simulink model "OPENXWD"  (R2021b)
settings: Solver=ode45  StartTime=0.0  StopTime=inf  RelTol=1e-3  EnableMultiTasking=on
PreLoadFcn:
  | run('Parameters\FSE_Parameters.m')
undefined symbols (not defined in the file): i_Diff
libraries: simulink x28, CarMaker4SL x17, eeGeneralControl x6
(part 3 of 8)

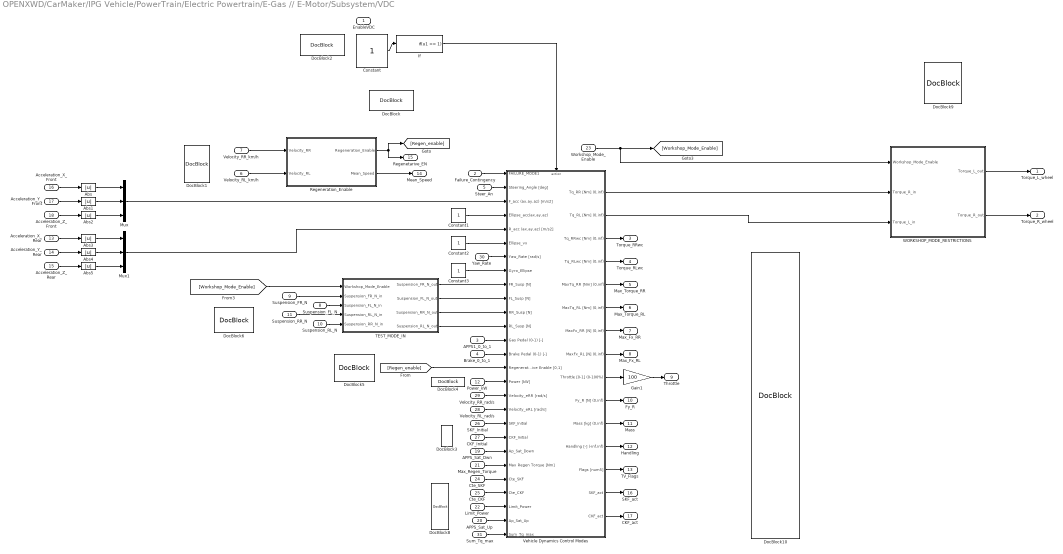
== system OPENXWD/CarMaker/IPG Vehicle/PowerTrain/Electric Powertrain/E-Gas // E-Motor/Subsystem/VDC ==
  EnableVDC : Inport
  Failure_Contingency : Inport  Port=2
  APPS1_0_to_1 : Inport  Port=3
  Brake_0_to_1 : Inport  Port=4
  Steer_An : Inport  Port=5
  Velocity_RL_km/h : Inport  Port=6
  Velocity_RR_km/h : Inport  Port=7
  Suspension_FL_N : Inport  Port=8
  Suspension_FR_N : Inport  Port=9
  Suspension_RL_N : Inport  Port=10
  Suspension_RR_N : Inport  Port=11
  Power_kW : Inport  Port=12
  Acceleration_X_Rear : Inport  Port=13
  Acceleration_Y_Rear : Inport  Port=14
  Acceleration_Z_Rear : Inport  Port=15
  Acceleration_X_Front : Inport  Port=16
  Acceleration_Y_Front : Inport  Port=17
  Acceleration_Z_Front : Inport  Port=18
  APPS_Sat_Dwn : Inport  Port=19
  APPS_Sat_Up : Inport  Port=20
  Max_Regen_Torque : Inport  Port=21
  Limit_Power : Inport  Port=22
  Workshop_Mode_Enable : Inport  Port=23
  Cte_SKF : Inport  Port=24
  Cte_CKF : Inport  Port=25
  SKF_Initial : Inport  Port=26
  CKF_Initial : Inport  Port=27
  Velocity_RL_rad/s : Inport  Port=28
  Velocity_RR_rad/s : Inport  Port=29
  Yaw_Rate : Inport  Port=30
  Sum_Tq_max : Inport  Port=31
  Abs{,1..5} (6 alike) : Abs
  Constant{,1..3} (4 alike) : Constant
  DocBlock{,1..6,8..10} (10 alike) : simulink/Model-Wide Utilities/DocBlock  DocumentType=Text
  Gain1 : Gain  Gain=100
  If : If  IfExpression=u1 == 1  ShowElse=off
  Mux : Mux  Inputs=3
  Mux1 : Mux  Inputs=3
  Regeneration_Enable : Subsystem  TreatAsAtomicUnit=on
  TEST_MODE_IN : Subsystem  TreatAsAtomicUnit=on
  Vehicle Dynamics Control Modes : Subsystem
  WORKSHOP_MODE_RESTRICTIONS : Subsystem  TreatAsAtomicUnit=on
  Torque_L_wheel : Outport  VectorParamsAs1DForOutWhenUnconnected=off
  Torque_R_wheel : Outport  Port=2  VectorParamsAs1DForOutWhenUnconnected=off
  Torque_RRwc : Outport  Port=3  VectorParamsAs1DForOutWhenUnconnected=off
  Torque_RLwc : Outport  Port=4  VectorParamsAs1DForOutWhenUnconnected=off
  Max_Torque_RR : Outport  Port=5  VectorParamsAs1DForOutWhenUnconnected=off
  Max_Torque_RL : Outport  Port=6  VectorParamsAs1DForOutWhenUnconnected=off
  Max_Fx_RR : Outport  Port=7  VectorParamsAs1DForOutWhenUnconnected=off
  Max_Fx_RL : Outport  Port=8  VectorParamsAs1DForOutWhenUnconnected=off
  Throttle : Outport  Port=9  VectorParamsAs1DForOutWhenUnconnected=off
  Fy_R : Outport  Port=10  VectorParamsAs1DForOutWhenUnconnected=off
  Mass : Outport  Port=11  VectorParamsAs1DForOutWhenUnconnected=off
  Handling : Outport  Port=12  VectorParamsAs1DForOutWhenUnconnected=off
  TV_Flags : Outport  Port=13  VectorParamsAs1DForOutWhenUnconnected=off
  Mean_Speed : Outport  Port=14  VectorParamsAs1DForOutWhenUnconnected=off
  Regenetarive_EN : Outport  Port=15  VectorParamsAs1DForOutWhenUnconnected=off
  SKF_act : Outport  Port=16  VectorParamsAs1DForOutWhenUnconnected=off
  CKF_act : Outport  Port=17  VectorParamsAs1DForOutWhenUnconnected=off
  wires:
  Velocity_RR_km/h/1 -> Regeneration_Enable/1(Velocity_RR)
  Acceleration_Z_Front/1 -> Abs2/1
  Abs2/1 -> Mux/3
  Gain1/1 -> Throttle/1
  Vehicle Dynamics Control Modes/7(MaxFx_RR [N] (0,inf)) -> Max_Fx_RR/1
  Vehicle Dynamics Control Modes/6(MaxTq_RL [Nm] (0,inf)) -> Max_Torque_RL/1
  Acceleration_X_Rear/1 -> Abs3/1
  Acceleration_Y_Front/1 -> Abs1/1
  Abs4/1 -> Mux1/2
  Vehicle Dynamics Control Modes/8(MaxFx_RL [N] (0,inf)) -> Max_Fx_RL/1
  Power_kW/1 -> Vehicle Dynamics Control Modes/16(Power [kW])
  Vehicle Dynamics Control Modes/1(Tq_RR [Nm] (0,inf)) -> WORKSHOP_MODE_RESTRICTIONS/2(Torque_R_in)
  Abs/1 -> Mux/1
  Abs5/1 -> Mux1/3
  Acceleration_Y_Rear/1 -> Abs4/1
  APPS_Sat_Up/1 -> Vehicle Dynamics Control Modes/26(Ap_Sat_Up)
  WORKSHOP_MODE_RESTRICTIONS/1(Torque_L_out) -> Torque_L_wheel/1
  Acceleration_Z_Rear/1 -> Abs5/1
  Vehicle Dynamics Control Modes/3(Tq_RRwc [Nm] (0,inf)) -> Torque_RRwc/1
  Suspension_FL_N/1 -> TEST_MODE_IN/3(Suspension_FL_N_in)
  Suspension_FR_N/1 -> TEST_MODE_IN/2(Suspension_FR_N_in)
  TEST_MODE_IN/1(Suspension_FR_N_out) -> Vehicle Dynamics Control Modes/9(FR_Susp [N])
  Velocity_RR_rad/s/1 -> Vehicle Dynamics Control Modes/17(Velocity_eRR [rad/s])
  Vehicle Dynamics Control Modes/14(SKF_act) -> SKF_act/1
  APPS1_0_to_1/1 -> Vehicle Dynamics Control Modes/13(Gas Pedal (0-1) [-])
  Vehicle Dynamics Control Modes/4(Tq_RLwc [Nm] (0,inf)) -> Torque_RLwc/1
  Vehicle Dynamics Control Modes/5(MaxTq_RR [Nm] (0,inf)) -> Max_Torque_RR/1
  Brake_0_to_1/1 -> Vehicle Dynamics Control Modes/14(Brake Pedal (0-1) [-])
  Velocity_RL_km/h/1 -> Regeneration_Enable/2(Velocity_RL)
  Vehicle Dynamics Control Modes/11(Mass [kg] (0,inf)) -> Mass/1
  Vehicle Dynamics Control Modes/9(Throttle [0-1] (0-100%)) -> Gain1/1
  Vehicle Dynamics Control Modes/2(Tq_RL [Nm] (0,inf)) -> WORKSHOP_MODE_RESTRICTIONS/3(Torque_L_in)
  Constant/1 -> If/1
  Regeneration_Enable/2(Mean_Speed) -> Mean_Speed/1
  Suspension_RL_N/1 -> TEST_MODE_IN/5(Suspension_RR_N_in)
  Vehicle Dynamics Control Modes/10(Fy_R [N] (0,inf)) -> Fy_R/1
  Vehicle Dynamics Control Modes/13(Flags [num5]) -> TV_Flags/1
  Abs1/1 -> Mux/2
  [Workshop_Mode_Enable] -> TEST_MODE_IN/1(Workshop_Mode_Enable)
  Acceleration_X_Front/1 -> Abs/1
  Abs3/1 -> Mux1/1
  Suspension_RR_N/1 -> TEST_MODE_IN/4(Suspension_RL_N_in)
  Vehicle Dynamics Control Modes/12(Handling [-] (-inf,inf)) -> Handling/1
  Workshop_Mode_Enable/1 -> [Workshop_Mode_Enable], WORKSHOP_MODE_RESTRICTIONS/1(Workshop_Mode_Enable)
  Vehicle Dynamics Control Modes/15(CKF_act) -> CKF_act/1
  If/1 -> Vehicle Dynamics Control Modes/Action
  TEST_MODE_IN/2(Suspension_FL_N_out) -> Vehicle Dynamics Control Modes/10(FL_Susp [N])
  TEST_MODE_IN/3(Suspension_RR_N_out) -> Vehicle Dynamics Control Modes/11(RR_Susp [N])
  TEST_MODE_IN/4(Suspension_RL_N_out) -> Vehicle Dynamics Control Modes/12(RL_Susp [N])
  Velocity_RL_rad/s/1 -> Vehicle Dynamics Control Modes/18(Velocity_eRL [rad/s])
  SKF_Initial/1 -> Vehicle Dynamics Control Modes/19(SKF_Initial)
  CKF_Initial/1 -> Vehicle Dynamics Control Modes/20(CKF_Initial)
  APPS_Sat_Dwn/1 -> Vehicle Dynamics Control Modes/21(Ap_Sat_Down)
  Max_Regen_Torque/1 -> Vehicle Dynamics Control Modes/22(Max Regen Torque [Nm])
  Cte_SKF/1 -> Vehicle Dynamics Control Modes/23(Cte_SKF)
  Cte_CKF/1 -> Vehicle Dynamics Control Modes/24(Cte_CKF)
  Steer_An/1 -> Vehicle Dynamics Control Modes/2(Steering_Angle [deg])
  Mux/1 -> Vehicle Dynamics Control Modes/3(F_acc (ax,ay,az) [m/s2])
  Mux1/1 -> Vehicle Dynamics Control Modes/5(R_acc (ax,ay,az) [m/s2])
  Failure_Contingency/1 -> Vehicle Dynamics Control Modes/1(FAILURE_MODE1)
  Constant1/1 -> Vehicle Dynamics Control Modes/4(Ellipse_acc(ax,ay,az))
  Constant2/1 -> Vehicle Dynamics Control Modes/6(Ellipse_vx)
  Yaw_Rate/1 -> Vehicle Dynamics Control Modes/7(Yaw_Rate [rad/s])
  Constant3/1 -> Vehicle Dynamics Control Modes/8(Gyro_Ellipse)
  Regeneration_Enable/1(Regeneration_Enable) -> Regenetarive_EN/1, [Regen_enable]
  [Regen_enable] -> Vehicle Dynamics Control Modes/15(Regenerative Enable [0,1])
  WORKSHOP_MODE_RESTRICTIONS/2(Torque_R_out) -> Torque_R_wheel/1
  Limit_Power/1 -> Vehicle Dynamics Control Modes/25(Limit_Power)
  Sum_Tq_max/1 -> Vehicle Dynamics Control Modes/27(Sum_Tq_max)

== system OPENXWD/CarMaker/IPG Vehicle/PowerTrain/Electric Powertrain/E-Gas // E-Motor/Subsystem/W to kW ==
  Power : Inport
  0-100 to 0-2 : Constant  Value=1000
  Divide5 : Product  Inputs=*/
  Out : Outport  VectorParamsAs1DForOutWhenUnconnected=off
  wires:
  Power/1 -> Divide5/1
  0-100 to 0-2/1 -> Divide5/2
  Divide5/1 -> Out/1

== system OPENXWD/CarMaker/IPG Vehicle/PowerTrain/Electric Powertrain/E-Gas // E-Motor/Subsystem/power_limitation1 ==
  note: Inputs:
      | max_cell_temp: signal from AMS_Master (Highest_Cell_Temp) [ºC]
      | max_inverter_temp: highest temperature of any of the inverters [ºC]
      | max_motor_temp: highest temperature of any of the motors [ºC]
      | SoC_Low, SoC_High: Lowest & Highest cell state of charge (0-100) [%]
  note: Outputs:
      | Flags: 1 means power is being limited by temperature, 0 means not limited
      | SoP_discharge: State of Power for discharging
      | SoP_charge: State of Power for charging
  max_motor_temp : Inport
  max_inverter_temp : Inport  Port=2
  max_cell_temp : Inport  Port=3
  SoC_Low : Inport  Port=4
  SoC_High : Inport  Port=5
  Saturation : Saturate  UpperLimit=1  LowerLimit=0
  Saturation1 : Saturate  UpperLimit=1  LowerLimit=0
  SoC_SoP : Subsystem
  initial_limitation : Constant  Value=0.4
  temperature_SoP : Subsystem
  Accu_Temperature_Limitation_Flag : Outport
  Inverters_Temperature_Limitation_Flag : Outport  Port=2
  Motors_Temperature_Limitation_Flag : Outport  Port=3
  SoP_Discharge : Outport  Port=4
  SoP_Regen : Outport  Port=5
  wires:
  SoC_SoP/1(SoP_Discharge) -> Saturation/1  "SoP_Discharge"
  SoC_SoP/2(SoP_Regen) -> Saturation1/1  "SoP_Regen"
  max_motor_temp/1 -> temperature_SoP/1(max_motor_temp)
  max_inverter_temp/1 -> temperature_SoP/2(max_inverter_temp)
  max_cell_temp/1 -> temperature_SoP/3(max_cell_temp), SoC_SoP/4(max_cell_temp)
  initial_limitation/1 -> temperature_SoP/4(initial_limitation)
  temperature_SoP/1(SoP) -> SoC_SoP/3(SoP_Temperature)  "temperature_SoP"
  temperature_SoP/4(Motors_Temperature_Limitation_Flag) -> Motors_Temperature_Limitation_Flag/1
  temperature_SoP/3(Inverters_Temperature_Limitation_Flag) -> Inverters_Temperature_Limitation_Flag/1
  temperature_SoP/2(Accu_Temperature_Limitation_Flag) -> Accu_Temperature_Limitation_Flag/1
  SoC_High/1 -> SoC_SoP/2(SoC_High)
  SoC_Low/1 -> SoC_SoP/1(SoC_Low)
  Saturation/1 -> SoP_Discharge/1
  Saturation1/1 -> SoP_Regen/1

== system OPENXWD/CarMaker/IPG Vehicle/PowerTrain/Electric Powertrain/E-Gas // E-Motor/Subsystem/Accumulator Power/PowerLimitDetection ==
  note: mean:500ms
      | time:25ms
      | moving window: 500/25=20
  Power : Inport
  Data Store Memory10 : DataStoreMemory  ReadBeforeWriteMsg=warning  WriteAfterWriteMsg=warning  WriteAfterReadMsg=warning  ShowAdditionalParam=off
  Data Store Read30 : DataStoreRead  IndexOptions=Index vector (dialog)  Indices=1  OutputSizes=1
  Data Store Write20 : DataStoreWrite  IndexOptions=Index vector (dialog)  Indices=1  OutputSizes=1
  If : If  IfExpression=u1 >= 80000
  LimitReached : Subsystem  TreatAsAtomicUnit=on
  Merge1 : Merge
  OK_OrLatch : Subsystem  TreatAsAtomicUnit=on
  PowerLimitReached : Outport  VectorParamsAs1DForOutWhenUnconnected=off
  PowerMean500ms : Outport  Port=2  VectorParamsAs1DForOutWhenUnconnected=off
  wires:
  Power/1 -> If/1, PowerMean500ms/1
  If/1 -> LimitReached/Action
  If/2 -> OK_OrLatch/Action
  LimitReached/1("Out ") -> Merge1/1
  OK_OrLatch/1(Out 1) -> Merge1/2
  Merge1/1 -> Data Store Write20/1, PowerLimitReached/1
  Data Store Read30/1 -> OK_OrLatch/1(IN)

== system OPENXWD/CarMaker/IPG Vehicle/PowerTrain/Electric Powertrain/E-Gas // E-Motor/Subsystem/Calculate Current Conversion/KT_L_TORKY ==
  Torque : Inport
  A/Nm : Gain  Gain=0.2
  Current : Outport  VectorParamsAs1DForOutWhenUnconnected=off
  wires:
  A/Nm/1 -> Current/1
  Torque/1 -> A/Nm/1

== system OPENXWD/CarMaker/IPG Vehicle/PowerTrain/Electric Powertrain/E-Gas // E-Motor/Subsystem/Calculate Current Conversion/KT_R_EMY ==
  Torque : Inport
  A/Nm : Gain  Gain=0.2
  Current : Outport  VectorParamsAs1DForOutWhenUnconnected=off
  wires:
  Torque/1 -> A/Nm/1
  A/Nm/1 -> Current/1

== system OPENXWD/CarMaker/IPG Vehicle/PowerTrain/Electric Powertrain/E-Gas // E-Motor/Subsystem/Controls Temperature by limiting Torque/SoC_SoP ==
  note: El lookup se puede obtener ensayando una celda en una descarga y en una carga con pérdidas de calor constantes. La corriente normalizada será el lookup.
  note: Si está descargada, no descargues más
  note: Si está cargada, no
      | cargues más
  SoC_Low : Inport
  SoC_High : Inport  Port=2
  SoP_Temperature : Inport  Port=3
  max_cell_temp : Inport  Port=4
  Gain5 : Gain  Gain=1/100
  Gain6 : Gain  Gain=1/100
  Lookup_SoC_SoP_chg : Lookup_n-D  NumberOfTableDimensions=1  BreakpointsForDimension1=[0.02 0.1 0.2 0.3 0.5 0.8 0.95 1]  Table=[0.95 1 1 1 1 0.9 0.75 0.02]  InternalRulePriority=Speed  RndMeth=Simplest  InputSameDT=on
  Lookup_SoC_SoP_dischg : Lookup_n-D  NumberOfTableDimensions=1  BreakpointsForDimension1=[0.02 0.1 0.2 0.3 0.5 0.8 0.9 1]  Table=[0.4 0.6 0.8 0.95 1 1 0.98 0.95]  InternalRulePriority=Speed  RndMeth=Simplest  InputSameDT=on
  Lookup_Temp_SoP_chg : Lookup_n-D  NumberOfTableDimensions=1  BreakpointsForDimension1=[45 48 49 50 51]  Table=[1 0.75 0.5 0 0]  InternalRulePriority=Speed  RndMeth=Simplest  InputSameDT=on
  Product : Product
  Product4 : Product
  Product5 : Product
  SoP_Discharge : Outport
  SoP_Regen : Outport  Port=2
  wires:
  Lookup_SoC_SoP_dischg/1 -> Product4/1
  Product/1 -> Product5/2
  SoP_Temperature/1 -> Product4/2, Product5/1
  SoC_Low/1 -> Gain6/1
  Gain6/1 -> Lookup_SoC_SoP_dischg/1
  SoC_High/1 -> Gain5/1
  Gain5/1 -> Lookup_SoC_SoP_chg/1
  Product5/1 -> SoP_Regen/1
  Product4/1 -> SoP_Discharge/1
  Lookup_SoC_SoP_chg/1 -> Product/1
  max_cell_temp/1 -> Lookup_Temp_SoP_chg/1
  Lookup_Temp_SoP_chg/1 -> Product/2

== system OPENXWD/CarMaker/IPG Vehicle/PowerTrain/Electric Powertrain/E-Gas // E-Motor/Subsystem/Controls Temperature by limiting Torque/temperature_SoP ==
  max_motor_temp : Inport
  max_inverter_temp : Inport  Port=2
  max_cell_temp : Inport  Port=3
  initial_limitation : Inport  Port=4
  Flag_Accu : simulink/Logic and Bit Operations/Compare To Constant  relop=<  const=1  OutDataTypeStr=boolean  ZeroCross=off
  Flag_Inv : simulink/Logic and Bit Operations/Compare To Constant  relop=<  const=1  OutDataTypeStr=boolean  ZeroCross=off
  Flag_Mot : simulink/Logic and Bit Operations/Compare To Constant  relop=<  const=1  OutDataTypeStr=boolean  ZeroCross=off
  Min : MinMax  Inputs=3
  temperature_rise_limitator_Accu : Subsystem
  temperature_rise_limitator_Inverters : Subsystem
  temperature_rise_limitator_Motors : Subsystem
  SoP : Outport
  Accu_Temperature_Limitation_Flag : Outport  Port=2
  Inverters_Temperature_Limitation_Flag : Outport  Port=3
  Motors_Temperature_Limitation_Flag : Outport  Port=4
  wires:
  temperature_rise_limitator_Inverters/1(SoP) -> Flag_Inv/1, Min/2
  initial_limitation/1 -> temperature_rise_limitator_Accu/2(initial_limitation), temperature_rise_limitator_Motors/2(initial_limitation), temperature_rise_limitator_Inverters/2(initial_limitation)
  Flag_Accu/1 -> Accu_Temperature_Limitation_Flag/1
  temperature_rise_limitator_Motors/1(SoP) -> Flag_Mot/1, Min/3
  max_cell_temp/1 -> temperature_rise_limitator_Accu/1(max_cell_temp)
  temperature_rise_limitator_Accu/1(SoP) -> Flag_Accu/1, Min/1
  Min/1 -> SoP/1
  Flag_Inv/1 -> Inverters_Temperature_Limitation_Flag/1
  Flag_Mot/1 -> Motors_Temperature_Limitation_Flag/1
  max_inverter_temp/1 -> temperature_rise_limitator_Inverters/1(max_inverter_temp)
  max_motor_temp/1 -> temperature_rise_limitator_Motors/1(max_motor_temp)

== system OPENXWD/CarMaker/IPG Vehicle/PowerTrain/Electric Powertrain/E-Gas // E-Motor/Subsystem/Pumps_Controller/Pumps_Control_OFF ==
  Action Port : ActionPort  ActionPortLabel=else
  Constant : Constant  Value=0
  0 : Outport  VectorParamsAs1DForOutWhenUnconnected=off
  wires:
  Constant/1 -> 0/1

== system OPENXWD/CarMaker/IPG Vehicle/PowerTrain/Electric Powertrain/E-Gas // E-Motor/Subsystem/Pumps_Controller/Pumps_Control_ON ==
  Action Port : ActionPort  ActionPortLabel=if(u1 == 1)
  Constant : Constant
  1 : Outport  VectorParamsAs1DForOutWhenUnconnected=off
  wires:
  Constant/1 -> 1/1

== system OPENXWD/CarMaker/IPG Vehicle/PowerTrain/Electric Powertrain/E-Gas // E-Motor/Subsystem/SAFETY BLOCK/APPS_IMPLAUSIBILITY ==
  APPS1 : Inport
  APPS2 : Inport  Port=2
  Ab : Abs
  If : If  IfExpression=u1 > 0.25
  Imp : Subsystem  TreatAsAtomicUnit=on
  Merge : Merge
  Not Imp : Subsystem  TreatAsAtomicUnit=on
  Sum : Sum  Inputs=|+-
  OK : Outport  VectorParamsAs1DForOutWhenUnconnected=off
  wires:
  APPS1/1 -> Sum/1
  APPS2/1 -> Sum/2
  Sum/1 -> Ab/1
  Ab/1 -> If/1
  Imp/1(Out1) -> Merge/1  "Bool 0"
  Not Imp/1(Out1) -> Merge/2  "Bool 1"
  Merge/1 -> OK/1
  If/2 -> Not Imp/Action
  If/1 -> Imp/Action

== system OPENXWD/CarMaker/IPG Vehicle/PowerTrain/Electric Powertrain/E-Gas // E-Motor/Subsystem/SAFETY BLOCK/BRAKE_IMPLAUSIBILITY ==
  APPS1_Value : Inport
  APPS2_Value : Inport  Port=2
  BrakeSensor_Value : Inport  Port=3
  Data Store Memory1 : DataStoreMemory  DataStoreName=AA  ReadBeforeWriteMsg=warning  WriteAfterWriteMsg=warning  WriteAfterReadMsg=warning  ShowAdditionalParam=off
  Data Store Read1 : DataStoreRead  DataStoreName=AA  IndexOptions=Index vector (dialog)  Indices=1  OutputSizes=1
  Data Store Write1 : DataStoreWrite  DataStoreName=AA  IndexOptions=Index vector (dialog)  Indices=1  OutputSizes=1
  If Action Subsystem2 : Subsystem  TreatAsAtomicUnit=on
  If Action Subsystem3 : Subsystem  TreatAsAtomicUnit=on
  If2 : If  NumInputs=3  IfExpression=(u1 > 0.25 & u3 > 0.25)|(u2 > 0.25 & u3 > 0.25)
  If3 : If  IfExpression=u1
  Imp Memo1 : Subsystem  TreatAsAtomicUnit=on
  Imp1 : Subsystem  TreatAsAtomicUnit=on
  Logical Operator1 : Logic  OutDataTypeStr=boolean
  MEMO1 : If  NumInputs=3  IfExpression=(u1 == 0 & u2 >0.05)|(u1 == 0 & u3 >0.05)
  Merge3 : Merge
  Merge4 : Merge
  Merge5 : Merge
  Not Imp Memo1 : Subsystem  TreatAsAtomicUnit=on
  Not Imp1 : Subsystem  TreatAsAtomicUnit=on
  OK_BRS : Outport  VectorParamsAs1DForOutWhenUnconnected=off
  wires:
  Imp Memo1/1(Out1) -> Merge4/1  "Bool 0"
  Data Store Read1/1 -> If3/1
  Merge5/1 -> MEMO1/1
  If3/1 -> If Action Subsystem2/Action
  If Action Subsystem3/1(Out1) -> Merge5/2
  Imp1/1(Out1) -> Merge3/1  "Bool 0"
  If3/2 -> If Action Subsystem3/Action
  Not Imp Memo1/1(Out1) -> Merge4/2  "Bool 1"
  Not Imp1/1(Out1) -> Merge3/2  "Bool 1"
  If2/2 -> Not Imp1/Action
  If2/1 -> Imp1/Action
  MEMO1/2 -> Not Imp Memo1/Action
  Merge3/1 -> Logical Operator1/1
  BrakeSensor_Value/1 -> If2/3
  APPS2_Value/1 -> MEMO1/3, If2/2
  MEMO1/1 -> Imp Memo1/Action
  If Action Subsystem2/1(Out1) -> Merge5/1
  Merge4/1 -> Logical Operator1/2
  APPS1_Value/1 -> MEMO1/2, If2/1
  Logical Operator1/1 -> OK_BRS/1, Data Store Write1/1

== system OPENXWD/CarMaker/IPG Vehicle/PowerTrain/Electric Powertrain/E-Gas // E-Motor/Subsystem/VDC/Regeneration_Enable ==
  note: Regen is Enable if velocity is higher than 2 km/h, to avoid backwards velocity due to Regen Tq (negative)
  Velocity_RR : Inport
  Velocity_RL : Inport  Port=2
  Add : Sum
  Constant : Constant  Value=2
  Divide : Product  Inputs=*/
  Enabled : Constant
  "Enabled " : Subsystem  TreatAsAtomicUnit=on
  If : If  NumInputs=2  IfExpression=(u1>2)&(u2>2)
  Merge1 : Merge
  NotEnabled : Subsystem  TreatAsAtomicUnit=on
  "Zero " : Constant  Value=0
  Regeneration_Enable : Outport  VectorParamsAs1DForOutWhenUnconnected=off
  Mean_Speed : Outport  Port=2  VectorParamsAs1DForOutWhenUnconnected=off
  wires:
  Merge1/1 -> Regeneration_Enable/1
  Velocity_RR/1 -> Add/1, If/1
  Velocity_RL/1 -> Add/2, If/2
  If/1 -> "Enabled "/Action
  If/2 -> NotEnabled/Action
  "Zero "/1 -> NotEnabled/1(In1)
  Add/1 -> Divide/1
  Divide/1 -> Mean_Speed/1
  Constant/1 -> Divide/2
  NotEnabled/1(Out1) -> Merge1/2
  "Enabled "/1(Out1) -> Merge1/1
  Enabled/1 -> "Enabled "/1(In1)

== system OPENXWD/CarMaker/IPG Vehicle/PowerTrain/Electric Powertrain/E-Gas // E-Motor/Subsystem/VDC/TEST_MODE_IN ==
  Workshop_Mode_Enable : Inport
  Suspension_FR_N_in : Inport  Port=2
  Suspension_FL_N_in : Inport  Port=3
  Suspension_RL_N_in : Inport  Port=4
  Suspension_RR_N_in : Inport  Port=5
  BYPASS : Subsystem  TreatAsAtomicUnit=on
  If : If  IfExpression=u1 == 1
  Merge{,1..3} (4 alike) : Merge
  TEST_CONSTANTS : Subsystem  TreatAsAtomicUnit=on
  Suspension_FR_N_out : Outport  VectorParamsAs1DForOutWhenUnconnected=off
  Suspension_FL_N_out : Outport  Port=2  VectorParamsAs1DForOutWhenUnconnected=off
  Suspension_RR_N_out : Outport  Port=3  VectorParamsAs1DForOutWhenUnconnected=off
  Suspension_RL_N_out : Outport  Port=4  VectorParamsAs1DForOutWhenUnconnected=off
  wires:
  Suspension_FR_N_in/1 -> BYPASS/1(In1)
  Suspension_FL_N_in/1 -> BYPASS/2(In2)
  Suspension_RR_N_in/1 -> BYPASS/3(In3)
  Suspension_RL_N_in/1 -> BYPASS/4(In4)
  Merge/1 -> Suspension_FR_N_out/1
  Merge1/1 -> Suspension_FL_N_out/1
  Merge2/1 -> Suspension_RR_N_out/1
  Merge3/1 -> Suspension_RL_N_out/1
  BYPASS/1(Out1) -> Merge/1
  BYPASS/2(Out2) -> Merge1/1
  BYPASS/3(Out3) -> Merge2/1
  BYPASS/4(Out4) -> Merge3/1
  Workshop_Mode_Enable/1 -> If/1
  If/2 -> BYPASS/Action
  If/1 -> TEST_CONSTANTS/Action
  TEST_CONSTANTS/4(Out4) -> Merge3/2
  TEST_CONSTANTS/3(Out3) -> Merge2/2
  TEST_CONSTANTS/2(Out2) -> Merge1/2
  TEST_CONSTANTS/1(Out1) -> Merge/2

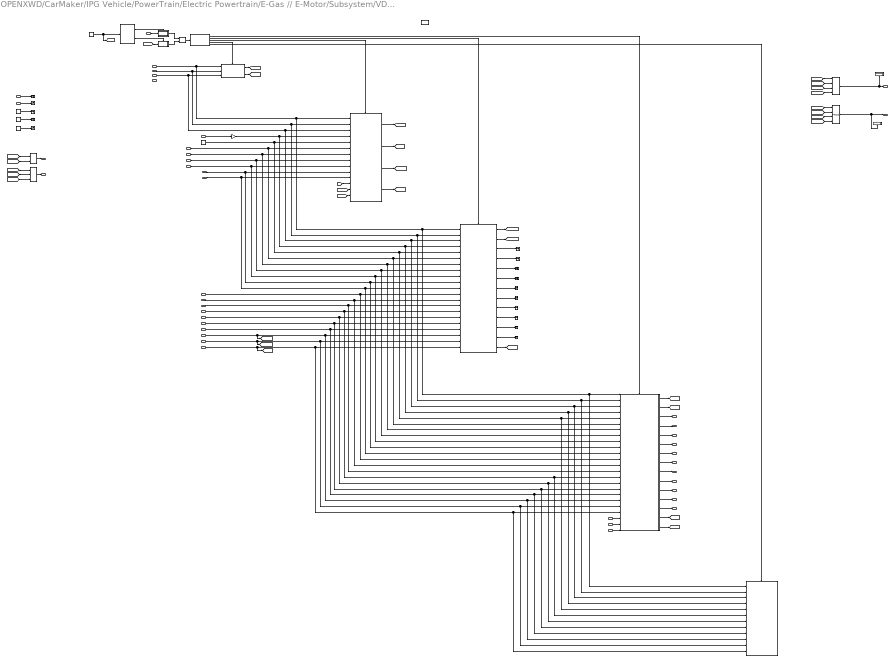
== system OPENXWD/CarMaker/IPG Vehicle/PowerTrain/Electric Powertrain/E-Gas // E-Motor/Subsystem/VDC/Vehicle Dynamics Control Modes ==
  note: CANVIAR A DISCONNECTIONS
  note: Failure Mode Selection: 4 -> Automatic Failure Mode Selection according to sensors available
      | 3 -> Rigid Axle (red)
      | 2 -> Steering TV with TC (orange)
      | 1 -> VDC without longitudinal (yellow)
      | 0-> VDC complete (green)
  note: Failure Mode Selection: 5 -> Automatic Failure Mode Selection according to sensors available
      | 4 -> Rigid Axle (red)
      | 3 -> Steering TV with TC (orange)
      | 2 -> VDC without longitudinal (yellow)
      | 1 -> VDC complete (green)
      | 0 -> TV with TC 2023
  FAILURE_MODE1 : Inport
  Steering_Angle [deg] : Inport  Port=2
  F_acc (ax,ay,az) [m/s2] : Inport  Port=3
  Ellipse_acc(ax,ay,az) : Inport  Port=4
  R_acc (ax,ay,az) [m/s2] : Inport  Port=5
  Ellipse_vx : Inport  Port=6
  Yaw_Rate [rad/s] : Inport  Port=7
  Gyro_Ellipse : Inport  Port=8
  FR_Susp [N] : Inport  Port=9
  FL_Susp [N] : Inport  Port=10
  RR_Susp [N] : Inport  Port=11
  RL_Susp [N] : Inport  Port=12
  Gas Pedal (0-1) [-] : Inport  Port=13
  Brake Pedal (0-1) [-] : Inport  Port=14
  Regenerative Enable [0,1] : Inport  Port=15
  Power [kW] : Inport  Port=16
  Velocity_eRR [rad/s] : Inport  Port=17
  Velocity_eRL [rad/s] : Inport  Port=18
  SKF_Initial : Inport  Port=19
  CKF_Initial : Inport  Port=20
  Ap_Sat_Down : Inport  Port=21
  Max Regen Torque [Nm] : Inport  Port=22
  Cte_SKF : Inport  Port=23
  Cte_CKF : Inport  Port=24
  Limit_Power : Inport  Port=25
  Ap_Sat_Up : Inport  Port=26
  Sum_Tq_max : Inport  Port=27
  Action Port : ActionPort  ActionPortLabel=if(u1 == 1)
  Automatic Failure Mode : Subsystem  TreatAsAtomicUnit=on
  Constant : Constant  Value=5
  Display : Display
  Display1 : Display
  FAILURE MODE : If  IfExpression=u1 == 1  ElseIfExpressions=u1 == 2, u1 == 3, u1 == 4, u1 == 0  ShowElse=off
  Gain : Gain  Gain=-1
  If : If  IfExpression=u1 == 5
  If Action Subsystem : Subsystem  TreatAsAtomicUnit=on
  Limit Temperature Celdas[ºC] : Constant  Value=45
  Limit Temperature IGBT [ºC] : Constant  Value=60
  Limit Temperature Motor [ºC] : Constant  Value=110
  Manual Failure Mode Selection : Subsystem  TreatAsAtomicUnit=on
  Merge : Merge
  Merge Tq_RL : Merge  Inputs=4
  Merge Tq_RR : Merge  Inputs=4
  Merge2 : Merge
  Merge3 : Merge  Inputs=3
  Rigid Axle : Subsystem  TreatAsAtomicUnit=on
  Steering TV with TC : Subsystem  TreatAsAtomicUnit=on
  "Steering Wheel Saturation (per site) [deg] " : Constant  Value=10
  Terminator{,1..14} (15 alike) : Terminator
  VDC Complete : Subsystem  TreatAsAtomicUnit=on
  VDC without Longitudinal : Subsystem  TreatAsAtomicUnit=on
  Tq_RR [Nm] (0,inf) : Outport  VectorParamsAs1DForOutWhenUnconnected=off
  Tq_RL [Nm] (0,inf) : Outport  Port=2  VectorParamsAs1DForOutWhenUnconnected=off
  Tq_RRwc [Nm] (0,inf) : Outport  Port=3  VectorParamsAs1DForOutWhenUnconnected=off
  Tq_RLwc [Nm] (0,inf) : Outport  Port=4  VectorParamsAs1DForOutWhenUnconnected=off
  MaxTq_RR [Nm] (0,inf) : Outport  Port=5  VectorParamsAs1DForOutWhenUnconnected=off
  MaxTq_RL [Nm] (0,inf) : Outport  Port=6  VectorParamsAs1DForOutWhenUnconnected=off
  MaxFx_RR [N] (0,inf) : Outport  Port=7  VectorParamsAs1DForOutWhenUnconnected=off
  MaxFx_RL [N] (0,inf) : Outport  Port=8  VectorParamsAs1DForOutWhenUnconnected=off
  Throttle [0-1] (0-100%) : Outport  Port=9  VectorParamsAs1DForOutWhenUnconnected=off
  Fy_R [N] (0,inf) : Outport  Port=10  VectorParamsAs1DForOutWhenUnconnected=off
  Mass [kg] (0,inf) : Outport  Port=11  VectorParamsAs1DForOutWhenUnconnected=off
  Handling [-] (-inf,inf) : Outport  Port=12  VectorParamsAs1DForOutWhenUnconnected=off
  Flags [num5] : Outport  Port=13  VectorParamsAs1DForOutWhenUnconnected=off
  SKF_act : Outport  Port=14  VectorParamsAs1DForOutWhenUnconnected=off
  CKF_act : Outport  Port=15  VectorParamsAs1DForOutWhenUnconnected=off
  wires:
  Ap_Sat_Up/1 -> Rigid Axle/1("Ap_Sat_up "), Steering TV with TC/1("Ap_Sat_up "), VDC without Longitudinal/1(Ap_Sat_Up [-]), If Action Subsystem/1(Ap_Sat_Up), VDC Complete/1(Ap_Sat_Up [-])
  VDC Complete/4(Tq_RLwc [Nm] (0,inf)) -> Tq_RLwc [Nm] (0,inf)/1
  VDC Complete/3(Tq_RRwc [Nm] (0,inf)) -> Tq_RRwc [Nm] (0,inf)/1
  VDC Complete/5(MaxTq_RR [Nm] (0,inf)) -> MaxTq_RR [Nm] (0,inf)/1
  VDC Complete/6(MaxTq_RL [Nm] (0,inf)) -> MaxTq_RL [Nm] (0,inf)/1
  VDC Complete/7(MaxFx_RR [N] (0,inf)) -> MaxFx_RR [N] (0,inf)/1
  VDC Complete/8(MaxFx_RL [N] (0,inf)) -> MaxFx_RL [N] (0,inf)/1
  VDC Complete/9(Throttle [0-1] (0-100%)) -> Throttle [0-1] (0-100%)/1
  VDC Complete/10(Fy_R [N] (0,inf)) -> Fy_R [N] (0,inf)/1
  VDC Complete/11(Mass [kg] (0,inf)) -> Mass [kg] (0,inf)/1
  VDC Complete/12(Handling [-] (-inf,inf)) -> Handling [-] (-inf,inf)/1
  VDC without Longitudinal/3(MaxTq_RR [Nm] (0,inf)) -> Terminator/1
  VDC without Longitudinal/4(MaxTq_RL [Nm] (0,inf)) -> Terminator1/1
  VDC without Longitudinal/5(MaxFx_RR [N] (0,inf)) -> Terminator2/1
  VDC without Longitudinal/6(MaxFx_RL [N] (0,inf)) -> Terminator3/1
  VDC without Longitudinal/7(Fy_R [N] (0,inf)) -> Terminator4/1
  VDC without Longitudinal/8(Throttle [0-1] (0-100%)) -> Terminator5/1
  VDC without Longitudinal/9(Mass [kg] (0,inf)) -> Terminator6/1
  VDC without Longitudinal/10(Handling [-] (-inf,inf)) -> Terminator7/1
  VDC without Longitudinal/11(Tq_RRwc [Nm] (0,inf)) -> Terminator8/1
  VDC without Longitudinal/12(Tq_RLwc [Nm] (0,inf)) -> Terminator9/1
  VDC Complete/13(Flags_[num5]) -> Flags [num5]/1
  Merge2/1 -> SKF_act/1
  Merge3/1 -> CKF_act/1
  Ap_Sat_Down/1 -> Steering TV with TC/2(Ap_Sat_down), If Action Subsystem/2(Ap_Sat_Down), VDC Complete/2(Ap_Sat_Down [-]), VDC without Longitudinal/2(Ap_Sat_Down [-]), Rigid Axle/2(Ap_Sat_down)
  Gas Pedal (0-1) [-]/1 -> Rigid Axle/3(Gas Pedal [0-1]), Steering TV with TC/3(Gas Pedal [0-1]), VDC without Longitudinal/3(Gas Pedal (0-1) [-]), If Action Subsystem/3(Gas Pedal), VDC Complete/3(Gas Pedal (0-1) [-])
  "Steering Wheel Saturation (per site) [deg] "/1 -> Steering TV with TC/5("Steering Wheel Saturation (per site) "), VDC without Longitudinal/5(Steering Saturation (per site) [deg]), If Action Subsystem/5(Steering saturation (per side) [deg]), VDC Complete/5(Steering Saturation (per site) [deg])
  SKF_Initial/1 -> VDC Complete/6(SKF_Initial), VDC without Longitudinal/6(SKF_initial), Steering TV with TC/6(SKF_Initial)
  CKF_Initial/1 -> VDC Complete/7(CKF_Initial), VDC without Longitudinal/7(CKF_Initial), Steering TV with TC/7(CKF_Initial)
  Cte_SKF/1 -> VDC Complete/8(Cte_SKF), VDC without Longitudinal/8(Cte_SKF), Steering TV with TC/8(Cte_SKF)
  Cte_CKF/1 -> VDC Complete/9(Cte_CKF), VDC without Longitudinal/9(Cte_CKF), Steering TV with TC/9(Cte_CKF)
  Velocity_eRL [rad/s]/1 -> Steering TV with TC/10(Vel_eRL), VDC Complete/10(Velocity_eRL [rad/s]), VDC without Longitudinal/10(Velocity_eRL [rad/s])
  Velocity_eRR [rad/s]/1 -> Steering TV with TC/11(Vel_eRR), VDC Complete/11(Velocity_eRR [rad/s]), VDC without Longitudinal/11(Velocity_eRR [rad/s])
  Steering TV with TC/3(SKF_act) -> [SKF_act2]
  Steering TV with TC/4(CKF_act) -> [CKF_act2]
  VDC without Longitudinal/13(CKF_act) -> [CKF_act1]
  VDC Complete/14(SKF_act) -> [SKF_act0]
  VDC Complete/15(CKF_act) -> [CKF_act0]
  [CKF_act1] -> Merge3/2
  [CKF_act0] -> Merge3/1
  [CKF_act2] -> Merge3/3
  [SKF_act0] -> Merge2/1
  [SKF_act2] -> Merge2/2
  Steering_Angle [deg]/1 -> Gain/1
  FAILURE MODE/1 -> VDC Complete/Action
  FAILURE MODE/2 -> VDC without Longitudinal/Action
  FAILURE MODE/3 -> Steering TV with TC/Action
  FAILURE MODE/4 -> Rigid Axle/Action
  Brake Pedal (0-1) [-]/1 -> If Action Subsystem/12(Brake Pedal), VDC Complete/21(Brake Pedal (0-1) [-]), VDC without Longitudinal/21(Brake Pedal (0-1) [-]), [Bp]
  F_acc (ax,ay,az) [m/s2]/1 -> VDC Complete/12(F_acc (ax,ay,az) [m/s2]), VDC without Longitudinal/12(F_acc (ax,ay,az) [m/s2])
  Ellipse_acc(ax,ay,az)/1 -> VDC Complete/14(Ellipse_acc), VDC without Longitudinal/14(Ellipse_acc_ax_ay_az)
  R_acc (ax,ay,az) [m/s2]/1 -> VDC Complete/13(R_acc (ax,ay,az) [m/s2]), VDC without Longitudinal/13(R_acc (ax,ay,az) [m/s2])
  FR_Susp [N]/1 -> If Action Subsystem/6(FR_Susp [N]), VDC Complete/15(FR_Susp [N]), VDC without Longitudinal/15(FR_Susp [N])
  FL_Susp [N]/1 -> If Action Subsystem/7(FL_Susp [N]), VDC Complete/16(FL_Susp [N]), VDC without Longitudinal/16(FL_Susp [N])
  RR_Susp [N]/1 -> If Action Subsystem/8(RR_Susp [N]), VDC Complete/17(RR_Susp [N]), VDC without Longitudinal/17(RR_Susp [N])
  RL_Susp [N]/1 -> If Action Subsystem/9(RL_Susp [N]), VDC Complete/18(RL_Susp [N]), VDC without Longitudinal/18(RL_Susp [N])
  Regenerative Enable [0,1]/1 -> [Regen_enable], If Action Subsystem/10(Regen_enable), VDC Complete/19(Regenerative Enable [0,1]), VDC without Longitudinal/19(Regenerative Enable [0,1])
  Max Regen Torque [Nm]/1 -> [Max_Regen_Tq], If Action Subsystem/11(Max_Regen_Tq (wheel Tq)), VDC Complete/20(Max Regen Torque [Nm]), VDC without Longitudinal/20(Max Regen Torque [Nm])
  Ellipse_vx/1 -> VDC Complete/24(Ellipse_vx)
  Gyro_Ellipse/1 -> VDC Complete/23(Gyro_Ellipse)
  Yaw_Rate [rad/s]/1 -> VDC Complete/22(Yaw_Rate [rad/s])
  Gain/1 -> Steering TV with TC/4(Steering_Angle [deg]), If Action Subsystem/4(Steering angle [deg]), VDC Complete/4(Steering_Angle [deg]), VDC without Longitudinal/4(Steering_Angle [deg])
  Steering TV with TC/1(Tq_RR_E2 [Nm] (0,inf)) -> [Tq_RR_E2]
  Steering TV with TC/2(Tq_RL_E2 [Nm] (0,inf)) -> [Tq_RL_E2]
  VDC without Longitudinal/1(Tq_RR_E1 [Nm] (0,inf)) -> [Tq_RR_E1]
  VDC Complete/1(Tq_RR_E0 [Nm] (0,inf)) -> [Tq_RR_E0]
  VDC Complete/2(Tq_RL_E0 [Nm] (0,inf)) -> [Tq_RL_E0]
  Merge Tq_RR/1 -> Display/1, Tq_RR [Nm] (0,inf)/1
  Rigid Axle/1(Tq_RR_E3 [Nm] (0,inf)) -> [Tq_RR_E3]
  Rigid Axle/2(Tq_RL_E3 [Nm] (0,inf)) -> [Tq_RL_E3]
  Merge Tq_RL/1 -> Display1/1, Tq_RL [Nm] (0,inf)/1
  [Tq_RR_E0] -> Merge Tq_RR/4
  [Tq_RR_E1] -> Merge Tq_RR/3
  [Tq_RR_E2] -> Merge Tq_RR/2
  [Tq_RR_E3] -> Merge Tq_RR/1
  [Tq_RL_E0] -> Merge Tq_RL/4
  [Tq_RL_E1] -> Merge Tq_RL/3
  [Tq_RL_E2] -> Merge Tq_RL/2
  [Tq_RL_E3] -> Merge Tq_RL/1
  Limit Temperature IGBT [ºC]/1 -> Terminator10/1
  Limit Temperature Motor [ºC]/1 -> Terminator11/1
  Limit Temperature Celdas[ºC]/1 -> Terminator12/1
  Power [kW]/1 -> Terminator13/1
  Limit_Power/1 -> Terminator14/1
  [Bp] -> Steering TV with TC/12(Bp)
  [Max_Regen_Tq] -> Steering TV with TC/13(Max_Regen_Tq)
  [Regen_enable] -> Steering TV with TC/14(Regen_enable)
  If/1 -> Automatic Failure Mode/Action
  FAILURE_MODE1/1 -> Automatic Failure Mode/1(In1)
  If/2 -> Manual Failure Mode Selection/Action
  Constant/1 -> [FM_select], If/1
  [FM_select] -> Manual Failure Mode Selection/1(In1)
  Merge/1 -> FAILURE MODE/1
  Automatic Failure Mode/1(Out1) -> Merge/1
  Manual Failure Mode Selection/1(Out1) -> Merge/2
  FAILURE MODE/5 -> If Action Subsystem/Action
  VDC without Longitudinal/2(Tq_RL_E1 [Nm] (0,inf)) -> [Tq_RL_E1]

== system OPENXWD/CarMaker/IPG Vehicle/PowerTrain/Electric Powertrain/E-Gas // E-Motor/Subsystem/VDC/WORKSHOP_MODE_RESTRICTIONS ==
  Workshop_Mode_Enable : Inport
  Torque_R_in : Inport  Port=2
  Torque_L_in : Inport  Port=3
  BYPASS : Subsystem  TreatAsAtomicUnit=on
  If : If  IfExpression=u1 == 1
  Merge : Merge
  Merge1 : Merge
  Saturation : Saturate  UpperLimit=580  LowerLimit=-580
  Saturation1 : Saturate  UpperLimit=580  LowerLimit=-580
  "Torque_Reduction " : Subsystem  TreatAsAtomicUnit=on
  Torque_L_out : Outport  VectorParamsAs1DForOutWhenUnconnected=off
  Torque_R_out : Outport  Port=2  VectorParamsAs1DForOutWhenUnconnected=off
  wires:
  If/2 -> BYPASS/Action
  If/1 -> "Torque_Reduction "/Action
  Workshop_Mode_Enable/1 -> If/1
  Torque_R_in/1 -> "Torque_Reduction "/1(In1), BYPASS/1(In1)
  Torque_L_in/1 -> "Torque_Reduction "/2(In2), BYPASS/2(In2)
  BYPASS/1(Out1) -> Merge/1
  BYPASS/2(Out2) -> Merge1/2
  "Torque_Reduction "/1(Out1) -> Merge/2
  "Torque_Reduction "/2(Out2) -> Merge1/1
  Merge/1 -> Saturation/1
  Merge1/1 -> Saturation1/1
  Saturation/1 -> Torque_R_out/1
  Saturation1/1 -> Torque_L_out/1

== system OPENXWD/CarMaker/IPG Vehicle/PowerTrain/Electric Powertrain/E-Gas // E-Motor/Subsystem/power_limitation1/SoC_SoP ==
  note: El lookup se puede obtener ensayando una celda en una descarga y en una carga con pérdidas de calor constantes. La corriente normalizada será el lookup.
  note: Si está descargada, no descargues más
  note: Si está cargada, no
      | cargues más
  SoC_Low : Inport
  SoC_High : Inport  Port=2
  SoP_Temperature : Inport  Port=3
  max_cell_temp : Inport  Port=4
  Gain5 : Gain  Gain=1/100
  Gain6 : Gain  Gain=1/100
  Lookup_SoC_SoP_chg : Lookup_n-D  NumberOfTableDimensions=1  BreakpointsForDimension1=[0.02 0.1 0.2 0.3 0.5 0.8 0.95 1]  Table=[0.95 1 1 1 1 0.9 0.75 0.02]  InternalRulePriority=Speed  RndMeth=Simplest  InputSameDT=on
  Lookup_SoC_SoP_dischg : Lookup_n-D  NumberOfTableDimensions=1  BreakpointsForDimension1=[0.02 0.1 0.2 0.3 0.5 0.8 0.9 1]  Table=[0.4 0.6 0.8 0.95 1 1 0.98 0.95]  InternalRulePriority=Speed  RndMeth=Simplest  InputSameDT=on
  Lookup_Temp_SoP_chg : Lookup_n-D  NumberOfTableDimensions=1  BreakpointsForDimension1=[45 48 49 50 51]  Table=[1 0.75 0.5 0 0]  InternalRulePriority=Speed  RndMeth=Simplest  InputSameDT=on
  Product : Product
  Product4 : Product
  Product5 : Product
  SoP_Discharge : Outport
  SoP_Regen : Outport  Port=2
  wires:
  Lookup_SoC_SoP_dischg/1 -> Product4/1
  Product/1 -> Product5/2
  SoP_Temperature/1 -> Product4/2, Product5/1
  SoC_Low/1 -> Gain6/1
  Gain6/1 -> Lookup_SoC_SoP_dischg/1
  SoC_High/1 -> Gain5/1
  Gain5/1 -> Lookup_SoC_SoP_chg/1
  Product5/1 -> SoP_Regen/1
  Product4/1 -> SoP_Discharge/1
  Lookup_SoC_SoP_chg/1 -> Product/1
  max_cell_temp/1 -> Lookup_Temp_SoP_chg/1
  Lookup_Temp_SoP_chg/1 -> Product/2

== system OPENXWD/CarMaker/IPG Vehicle/PowerTrain/Electric Powertrain/E-Gas // E-Motor/Subsystem/power_limitation1/temperature_SoP ==
  max_motor_temp : Inport
  max_inverter_temp : Inport  Port=2
  max_cell_temp : Inport  Port=3
  initial_limitation : Inport  Port=4
  Flag_Accu : simulink/Logic and Bit Operations/Compare To Constant  relop=<  const=1  OutDataTypeStr=boolean  ZeroCross=off
  Flag_Inv : simulink/Logic and Bit Operations/Compare To Constant  relop=<  const=1  OutDataTypeStr=boolean  ZeroCross=off
  Flag_Mot : simulink/Logic and Bit Operations/Compare To Constant  relop=<  const=1  OutDataTypeStr=boolean  ZeroCross=off
  Min : MinMax  Inputs=3
  temperature_rise_limitator_Accu : Subsystem
  temperature_rise_limitator_Inverters : Subsystem
  temperature_rise_limitator_Motors : Subsystem
  SoP : Outport
  Accu_Temperature_Limitation_Flag : Outport  Port=2
  Inverters_Temperature_Limitation_Flag : Outport  Port=3
  Motors_Temperature_Limitation_Flag : Outport  Port=4
  wires:
  temperature_rise_limitator_Inverters/1(SoP) -> Flag_Inv/1, Min/2
  initial_limitation/1 -> temperature_rise_limitator_Accu/2(initial_limitation), temperature_rise_limitator_Motors/2(initial_limitation), temperature_rise_limitator_Inverters/2(initial_limitation)
  Flag_Accu/1 -> Accu_Temperature_Limitation_Flag/1
  temperature_rise_limitator_Motors/1(SoP) -> Flag_Mot/1, Min/3
  max_cell_temp/1 -> temperature_rise_limitator_Accu/1(max_cell_temp)
  temperature_rise_limitator_Accu/1(SoP) -> Flag_Accu/1, Min/1
  Min/1 -> SoP/1
  Flag_Inv/1 -> Inverters_Temperature_Limitation_Flag/1
  Flag_Mot/1 -> Motors_Temperature_Limitation_Flag/1
  max_inverter_temp/1 -> temperature_rise_limitator_Inverters/1(max_inverter_temp)
  max_motor_temp/1 -> temperature_rise_limitator_Motors/1(max_motor_temp)

== system OPENXWD/CarMaker/IPG Vehicle/PowerTrain/Electric Powertrain/E-Gas // E-Motor/Subsystem/Accumulator Power/PowerLimitDetection/LimitReached ==
  Action Port : ActionPort  ActionPortLabel=if(u1 >= 80000)
  Constant : Constant
  "Out " : Outport  VectorParamsAs1DForOutWhenUnconnected=off
  wires:
  Constant/1 -> "Out "/1

== system OPENXWD/CarMaker/IPG Vehicle/PowerTrain/Electric Powertrain/E-Gas // E-Motor/Subsystem/Accumulator Power/PowerLimitDetection/OK_OrLatch ==
  IN : Inport
  Action Port : ActionPort  ActionPortLabel=else
  If : If  IfExpression=(u1>0)
  Latched Error : Subsystem  TreatAsAtomicUnit=on
  Merge : Merge
  OK : Subsystem  TreatAsAtomicUnit=on
  Out 1 : Outport  VectorParamsAs1DForOutWhenUnconnected=off
  wires:
  IN/1 -> If/1
  If/1 -> Latched Error/Action
  If/2 -> OK/Action
  Latched Error/1("Out ") -> Merge/1
  OK/1("Out ") -> Merge/2
  Merge/1 -> Out 1/1

== system OPENXWD/CarMaker/IPG Vehicle/PowerTrain/Electric Powertrain/E-Gas // E-Motor/Subsystem/Controls Temperature by limiting Torque/temperature_SoP/temperature_rise_limitator_Accu ==
  note: initial_limitation es una constante para la reducción inicial (de 0 a 1, más bajo significa que cambia
      | menos, más alto la limitación
      | inicial es más bestia).
  note: saturamos de 1 a 0 por si acaso
  note: magia chunga para
      | que los números cuadren
  note: Se limita la corriente en proporción
      | al ratio entre la temperatura actual y 50ºC
  note: output 0 si está por
      | debajo de 50ºC, 1 si está
      | por encima
  max_cell_temp : Inport
  initial_limitation : Inport  Port=2
  Add1 : Sum  Inputs=-+
  Add2 : Sum  Inputs=-++
  Add3 : Sum  Inputs=+-
  Constant1 : Constant  Value=45
  Constant2 : Constant  Value=5
  Constant3 : Constant
  Divide : Product  Inputs=*/
  Low-Pass Filter (Discrete or Continuous)1 : eeGeneralControl/Low-Pass Filter (Discrete or Continuous)  K=1  T=100  B=inf  A=-inf  init_option=Inherited from block input  x0=0  Ts=-1
  Product4 : Product
  Saturation1 : Saturate  UpperLimit=1  LowerLimit=0
  Temp higher than 50 : simulink/Logic and Bit Operations/Compare To Constant  relop=>=  const=50  OutDataTypeStr=boolean  ZeroCross=off
  SoP : Outport
  wires:
  Divide/1 -> Add3/1
  Constant3/1 -> Add2/3
  Constant1/1 -> Divide/1
  max_cell_temp/1 -> Add1/2, Temp higher than 50/1
  Temp higher than 50/1 -> Add2/1, Product4/2
  Constant2/1 -> Add1/1
  Product4/1 -> Add2/2
  Add2/1 -> Low-Pass Filter (Discrete or Continuous)1/1
  Add3/1 -> Product4/1
  Add1/1 -> Divide/2
  Saturation1/1 -> SoP/1
  initial_limitation/1 -> Add3/2
  Low-Pass Filter (Discrete or Continuous)1/1 -> Saturation1/1

== system OPENXWD/CarMaker/IPG Vehicle/PowerTrain/Electric Powertrain/E-Gas // E-Motor/Subsystem/Controls Temperature by limiting Torque/temperature_SoP/temperature_rise_limitator_Inverters ==
  note: output 0 si está por
      | debajo de 50ºC, 1 si está
      | por encima
  note: Se limita la corriente en proporción
      | al ratio entre la temperatura actual y 50ºC
  note: magia chunga para
      | que los números cuadren
  note: saturamos de 1 a 0 por si acaso
  note: initial_limitation es una constante para la reducción inicial (de 0 a 1, más bajo significa que cambia
      | menos, más alto la limitación
      | inicial es más bestia).
  max_inverter_temp : Inport
  initial_limitation : Inport  Port=2
  Add1 : Sum  Inputs=-+
  Add2 : Sum  Inputs=-++
  Add3 : Sum  Inputs=+-
  Constant1 : Constant  Value=45
  Constant2 : Constant  Value=5
  Constant3 : Constant
  Divide : Product  Inputs=*/
  Low-Pass Filter (Discrete or Continuous) : eeGeneralControl/Low-Pass Filter (Discrete or Continuous)  K=1  T=100  B=inf  A=-inf  init_option=Inherited from block input  x0=0  Ts=-1
  Product4 : Product
  Saturation1 : Saturate  UpperLimit=1  LowerLimit=0
  Temp higher than 50 : simulink/Logic and Bit Operations/Compare To Constant  relop=>=  const=50  OutDataTypeStr=boolean  ZeroCross=off
  SoP : Outport
  wires:
  Low-Pass Filter (Discrete or Continuous)/1 -> Saturation1/1
  initial_limitation/1 -> Add3/2
  Saturation1/1 -> SoP/1
  Add1/1 -> Divide/2
  Add3/1 -> Product4/1
  Add2/1 -> Low-Pass Filter (Discrete or Continuous)/1
  Product4/1 -> Add2/2
  Constant2/1 -> Add1/1
  Temp higher than 50/1 -> Product4/2, Add2/1
  max_inverter_temp/1 -> Temp higher than 50/1, Add1/2
  Constant1/1 -> Divide/1
  Constant3/1 -> Add2/3
  Divide/1 -> Add3/1

== system OPENXWD/CarMaker/IPG Vehicle/PowerTrain/Electric Powertrain/E-Gas // E-Motor/Subsystem/Controls Temperature by limiting Torque/temperature_SoP/temperature_rise_limitator_Motors ==
  note: initial_limitation es una constante para la reducción inicial (de 0 a 1, más bajo significa que cambia
      | menos, más alto la limitación
      | inicial es más bestia).
  note: saturamos de 1 a 0 por si acaso
  note: magia chunga para
      | que los números cuadren
  note: Se limita la corriente en proporción
      | al ratio entre la temperatura actual y 110ºC
  note: output 0 si está por
      | debajo de 110ºC, 1 si está
      | por encima
  max_motor_temp : Inport
  initial_limitation : Inport  Port=2
  Add1 : Sum  Inputs=-+
  Add2 : Sum  Inputs=-++
  Add3 : Sum  Inputs=+-
  Constant1 : Constant  Value=105
  Constant2 : Constant  Value=5
  Constant3 : Constant
  Divide : Product  Inputs=*/
  Low-Pass Filter (Discrete or Continuous) : eeGeneralControl/Low-Pass Filter (Discrete or Continuous)  K=1  T=100  B=inf  A=-inf  init_option=Inherited from block input  x0=0  Ts=-1
  Product4 : Product
  Saturation1 : Saturate  UpperLimit=1  LowerLimit=0
  Temp higher than 110 : simulink/Logic and Bit Operations/Compare To Constant  relop=>=  const=110  OutDataTypeStr=boolean  ZeroCross=off
  SoP : Outport
  wires:
  Divide/1 -> Add3/1
  Constant3/1 -> Add2/3
  Constant1/1 -> Divide/1
  max_motor_temp/1 -> Add1/2, Temp higher than 110/1
  Temp higher than 110/1 -> Add2/1, Product4/2
  Constant2/1 -> Add1/1
  Product4/1 -> Add2/2
  Add2/1 -> Low-Pass Filter (Discrete or Continuous)/1
  Add3/1 -> Product4/1
  Add1/1 -> Divide/2
  Saturation1/1 -> SoP/1
  initial_limitation/1 -> Add3/2
  Low-Pass Filter (Discrete or Continuous)/1 -> Saturation1/1

== system OPENXWD/CarMaker/IPG Vehicle/PowerTrain/Electric Powertrain/E-Gas // E-Motor/Subsystem/SAFETY BLOCK/APPS_IMPLAUSIBILITY/Imp ==
  Action Port : ActionPort  ActionPortLabel=if(u1 > 0.25)
  Constant : Constant  Value=0  OutDataTypeStr=boolean
  Out1 : Outport  VectorParamsAs1DForOutWhenUnconnected=off
  wires:
  Constant/1 -> Out1/1  "Boolean"

== system OPENXWD/CarMaker/IPG Vehicle/PowerTrain/Electric Powertrain/E-Gas // E-Motor/Subsystem/SAFETY BLOCK/APPS_IMPLAUSIBILITY/Not Imp ==
  Action Port : ActionPort  ActionPortLabel=else
  Constant : Constant  OutDataTypeStr=boolean
  Out1 : Outport  VectorParamsAs1DForOutWhenUnconnected=off
  wires:
  Constant/1 -> Out1/1  "Boolean"

== system OPENXWD/CarMaker/IPG Vehicle/PowerTrain/Electric Powertrain/E-Gas // E-Motor/Subsystem/SAFETY BLOCK/BRAKE_IMPLAUSIBILITY/If Action Subsystem2 ==
  Action Port : ActionPort  ActionPortLabel=if(u1)
  Constant : Constant
  Out1 : Outport  VectorParamsAs1DForOutWhenUnconnected=off
  wires:
  Constant/1 -> Out1/1

== system OPENXWD/CarMaker/IPG Vehicle/PowerTrain/Electric Powertrain/E-Gas // E-Motor/Subsystem/SAFETY BLOCK/BRAKE_IMPLAUSIBILITY/If Action Subsystem3 ==
  Action Port : ActionPort  ActionPortLabel=else
  Constant : Constant  Value=0
  Out1 : Outport  VectorParamsAs1DForOutWhenUnconnected=off
  wires:
  Constant/1 -> Out1/1

== system OPENXWD/CarMaker/IPG Vehicle/PowerTrain/Electric Powertrain/E-Gas // E-Motor/Subsystem/SAFETY BLOCK/BRAKE_IMPLAUSIBILITY/Imp Memo1 ==
  Action Port : ActionPort  ActionPortLabel=if((u1 == 0 & u2 >0.05)|(u1 == 0 & u3 >0.05))
  Constant : Constant  Value=0  OutDataTypeStr=boolean
  Out1 : Outport  VectorParamsAs1DForOutWhenUnconnected=off
  wires:
  Constant/1 -> Out1/1  "Boolean"

== system OPENXWD/CarMaker/IPG Vehicle/PowerTrain/Electric Powertrain/E-Gas // E-Motor/Subsystem/SAFETY BLOCK/BRAKE_IMPLAUSIBILITY/Imp1 ==
  Action Port : ActionPort  ActionPortLabel=if((u1 > 0.25 & u3 > 0.25)|(u2 > 0.25 & u3 > 0.25))
  Constant : Constant  Value=0  OutDataTypeStr=boolean
  Out1 : Outport  VectorParamsAs1DForOutWhenUnconnected=off
  wires:
  Constant/1 -> Out1/1  "Boolean"

== system OPENXWD/CarMaker/IPG Vehicle/PowerTrain/Electric Powertrain/E-Gas // E-Motor/Subsystem/SAFETY BLOCK/BRAKE_IMPLAUSIBILITY/Not Imp Memo1 ==
  Action Port : ActionPort  ActionPortLabel=else
  Constant : Constant  OutDataTypeStr=boolean
  Out1 : Outport  VectorParamsAs1DForOutWhenUnconnected=off
  wires:
  Constant/1 -> Out1/1  "Boolean"

== system OPENXWD/CarMaker/IPG Vehicle/PowerTrain/Electric Powertrain/E-Gas // E-Motor/Subsystem/SAFETY BLOCK/BRAKE_IMPLAUSIBILITY/Not Imp1 ==
  Action Port : ActionPort  ActionPortLabel=else
  Constant : Constant  OutDataTypeStr=boolean
  Out1 : Outport  VectorParamsAs1DForOutWhenUnconnected=off
  wires:
  Constant/1 -> Out1/1  "Boolean"

== system OPENXWD/CarMaker/IPG Vehicle/PowerTrain/Electric Powertrain/E-Gas // E-Motor/Subsystem/VDC/Regeneration_Enable/Enabled  ==
  In1 : Inport
  Action Port : ActionPort  ActionPortLabel=if((u1>2)&(u2>2))
  Out1 : Outport  VectorParamsAs1DForOutWhenUnconnected=off
  wires:
  In1/1 -> Out1/1

== system OPENXWD/CarMaker/IPG Vehicle/PowerTrain/Electric Powertrain/E-Gas // E-Motor/Subsystem/VDC/Regeneration_Enable/NotEnabled ==
  In1 : Inport
  Action Port : ActionPort  ActionPortLabel=else
  Out1 : Outport  VectorParamsAs1DForOutWhenUnconnected=off
  wires:
  In1/1 -> Out1/1

== system OPENXWD/CarMaker/IPG Vehicle/PowerTrain/Electric Powertrain/E-Gas // E-Motor/Subsystem/VDC/TEST_MODE_IN/BYPASS ==
  In1 : Inport
  In2 : Inport  Port=2
  In3 : Inport  Port=3
  In4 : Inport  Port=4
  Action Port : ActionPort  ActionPortLabel=else
  Out1 : Outport  VectorParamsAs1DForOutWhenUnconnected=off
  Out2 : Outport  Port=2  VectorParamsAs1DForOutWhenUnconnected=off
  Out3 : Outport  Port=3  VectorParamsAs1DForOutWhenUnconnected=off
  Out4 : Outport  Port=4  VectorParamsAs1DForOutWhenUnconnected=off
  wires:
  In1/1 -> Out1/1
  In2/1 -> Out2/1
  In3/1 -> Out3/1
  In4/1 -> Out4/1

== system OPENXWD/CarMaker/IPG Vehicle/PowerTrain/Electric Powertrain/E-Gas // E-Motor/Subsystem/VDC/TEST_MODE_IN/TEST_CONSTANTS ==
  Action Port : ActionPort  ActionPortLabel=if(u1 == 1)
  Constant{,1..3} (4 alike) : Constant  Value=800
  Out1 : Outport  VectorParamsAs1DForOutWhenUnconnected=off
  Out2 : Outport  Port=2  VectorParamsAs1DForOutWhenUnconnected=off
  Out3 : Outport  Port=3  VectorParamsAs1DForOutWhenUnconnected=off
  Out4 : Outport  Port=4  VectorParamsAs1DForOutWhenUnconnected=off
  wires:
  Constant/1 -> Out1/1
  Constant1/1 -> Out2/1
  Constant2/1 -> Out3/1
  Constant3/1 -> Out4/1

== system OPENXWD/CarMaker/IPG Vehicle/PowerTrain/Electric Powertrain/E-Gas // E-Motor/Subsystem/VDC/Vehicle Dynamics Control Modes/Automatic Failure Mode ==
  In1 : Inport
  Action Port : ActionPort  ActionPortLabel=if(u1 == 5)
  Out1 : Outport  VectorParamsAs1DForOutWhenUnconnected=off
  wires:
  In1/1 -> Out1/1

== system OPENXWD/CarMaker/IPG Vehicle/PowerTrain/Electric Powertrain/E-Gas // E-Motor/Subsystem/VDC/Vehicle Dynamics Control Modes/If Action Subsystem ==
  Ap_Sat_Up : Inport
  Ap_Sat_Down : Inport  Port=2
  Gas Pedal : Inport  Port=3
  Steering angle [deg] : Inport  Port=4
  Steering saturation (per side) [deg] : Inport  Port=5
  FR_Susp [N] : Inport  Port=6
  FL_Susp [N] : Inport  Port=7
  RR_Susp [N] : Inport  Port=8
  RL_Susp [N] : Inport  Port=9
  Regen_enable : Inport  Port=10
  Max_Regen_Tq (wheel Tq) : Inport  Port=11
  Brake Pedal : Inport  Port=12
  Action Port : ActionPort  ActionPortLabel=elseif( u1 == 0)
  Max_Slip_RL : MATLAB Function  TreatAsAtomicUnit=on
  Max_Slip_RR : MATLAB Function  TreatAsAtomicUnit=on
  wires:
  RR_Susp [N]/1 -> Max_Slip_RR/1(Fz_RR)
  RL_Susp [N]/1 -> Max_Slip_RL/1(Fz_RL)

== system OPENXWD/CarMaker/IPG Vehicle/PowerTrain/Electric Powertrain/E-Gas // E-Motor/Subsystem/VDC/Vehicle Dynamics Control Modes/Manual Failure Mode Selection ==
  In1 : Inport
  Action Port : ActionPort  ActionPortLabel=else
  Out1 : Outport  VectorParamsAs1DForOutWhenUnconnected=off
  wires:
  In1/1 -> Out1/1

== system OPENXWD/CarMaker/IPG Vehicle/PowerTrain/Electric Powertrain/E-Gas // E-Motor/Subsystem/VDC/Vehicle Dynamics Control Modes/Rigid Axle ==
  "Ap_Sat_up " : Inport
  Ap_Sat_down : Inport  Port=2
  Gas Pedal [0-1] : Inport  Port=3
  Action Port : ActionPort  ActionPortLabel=elseif( u1 == 4)
  Accelerating : Subsystem
  RT_L : Gain  Gain=4
  RT_R : Gain  Gain=4
  Torque_RL [Nm] : Constant  Value=60
  Torque_RR [Nm] : Constant  Value=60
  Tq_RR_E3 [Nm] (0,inf) : Outport  VectorParamsAs1DForOutWhenUnconnected=off
  Tq_RL_E3 [Nm] (0,inf) : Outport  Port=2  VectorParamsAs1DForOutWhenUnconnected=off
  wires:
  Torque_RR [Nm]/1 -> RT_R/1
  Torque_RL [Nm]/1 -> RT_L/1
  Accelerating/2(Tq_RL) -> Tq_RL_E3 [Nm] (0,inf)/1
  Accelerating/1("Tq_RR ") -> Tq_RR_E3 [Nm] (0,inf)/1
  Gas Pedal [0-1]/1 -> Accelerating/1(Ap)
  "Ap_Sat_up "/1 -> Accelerating/2("Ap_Sat_up ")
  Ap_Sat_down/1 -> Accelerating/3(Ap_Sat_down)
  RT_R/1 -> Accelerating/4(Tq_RR)
  RT_L/1 -> Accelerating/5("Tq_RL ")
